simulink model "LAP_2018a"  (R2018a)
settings: Solver=VariableStepAuto  StartTime=0.0  StopTime=10.0  RelTol=1e-3
settings Model: Creator=apple  LastModifiedBy=apple
settings DataIOCC: ReturnWorkspaceOutputs=on
settings SFSimCC: SimUseLocalCustomCode=on
settings RTWCC: RTWUseLocalCustomCode=on

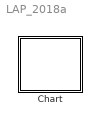
== system LAP_2018a ==
  Chart : Stateflow chart  TreatAsAtomicUnit=on

== stateflow chart LAP_2018a/Chart ==
  state RunW
    en:fprintf("en_RunW");
    state Running
      du:fprintf("edu_Running");
      disp_cent = cent;
      disp_sec = sec;
      disp_min = mins;
    state Lap
      en:fprintf("en_Lap");
    RunW -> (junction 29) : TIC{fprintf("cond_TIC");
        | cent = cent + 1;}
    (default) -> Running
    (junction 29) -> (junction 30) [order 1] : [cent == 100]{cent = 0;
        | sec = sec + 1;}
    (junction 29) -> (junction 31) [order 2]
    (junction 30) -> (junction 31) [order 2]
    (junction 30) -> (junction 31) [order 1] : [sec == 60]{sec = 0;
        | mins = mins + 1;}
    Running -> Lap [order 1] : LAP
    Lap -> Running [order 1] : LAP
  state StopW
    en:fprintf("en_StopW");
    state Reset
      en:fprintf("en_Reset");send(LAP);send(START);
      Reset -> (junction 16) [order 1] : LAP{cent = 0;sec=0;mins=0;
          | disp_cent=0;disp_sec=0;
          | disp_min=0;}
    state LapStop
      en:fprintf("en_LapStop");
    (default) -> Reset
    LapStop -> Reset [order 1] : LAP
  (default) -> StopW
  Reset -> Running [order 1] : START
  Running -> Reset [order 2] : START
  LapStop -> Lap [order 2] : START
  Lap -> LapStop [order 2] : START
  data: cent local; disp_min local; disp_cent local; disp_sec local; mins local; sec local
  events: LAP local FUNCTION_CALL_EVENT; START local FUNCTION_CALL_EVENT; TIC local FUNCTION_CALL_EVENT
